simulink model "Retroacao_de_estados_2a_Lei_simulink"  (R2019a)
settings: Solver=ode45  StartTime=0.0  StopTime=2  RelTol=1e-3  EnableMultiTasking=on
values from neighbouring files (symbols this model uses):
  a = [-1 1; 1 -2]    [Ganhos_observador_de_estados.m]    (also in Observador_de_estados.m; Retroacao_de_estados_1a_Lei.m = [0 1; -40 -3]; Retroacao_de_estados_2a_Lei.m = [[0 1]; [0 -50]])
  b = [1;0]    [Ganhos_observador_de_estados.m]    (also in Observador_de_estados.m; Retroacao_de_estados_1a_Lei.m = [0 ; 40]; Retroacao_de_estados_2a_Lei.m = [0;1370])
  c = [1 0]    [Ganhos_observador_de_estados.m]    (also in Observador_de_estados.m; Retroacao_de_estados_2a_Lei.m = eye(2))
  d = 0    [Retroacao_de_estados_2a_Lei.m]
  K1 = K(1)    [Retroacao_de_estados_1a_Lei.m]    (also in Retroacao_de_estados_2a_Lei.m; Retroacao_de_estados_3a_Lei.m)
  K2 = K(2)    [Retroacao_de_estados_1a_Lei.m]    (also in Retroacao_de_estados_2a_Lei.m)
settings Model: Creator=Joao Paulo  LastModifiedBy=vinic
settings DataIOCC: LimitDataPoints=on  SaveFormat=Array  ReturnWorkspaceOutputs=off
settings OptimizationCC: ExpressionDepthLimit=2147483647  LifeSpan=inf
settings DebuggingCC: UnderspecifiedInitializationDetection=Classic  MergeDetectMultiDrivingBlocksExec=none  SolverPrmCheckMsg=warning  AllowSymbolicDim=off  StateNameClashWarn=warning  SFUnexpectedBacktrackingDiag=warning  SFNoUnconditionalDefaultTransitionDiag=warning  SFExecutionAtInitializationDiag=none  ArithmeticOperatorsInVariantConditions=warning
settings HardwareCC: ProdBitPerPointer=32  ProdBitPerSizeT=32  ProdBitPerPtrDiffT=32  ProdLargestAtomicFloat=None  ProdIntDivRoundTo=Undefined  ProdEndianess=Unspecified  ProdWordSize=32  ProdHWDeviceType=32-bit Generic
settings ModelReferenceCC: PropagateSignalLabelsOutOfModel=off
settings SFSimCC: SimUseLocalCustomCode=off
settings RTWCC: RTWUseLocalCustomCode=off
settings CodeAppCC: StateflowObjectComments=on
settings GRTTargetCC: TargetLangStandard=C89/C90 (ANSI)  GeneratePreprocessorConditionals=Disable all
settings ConfigComp: CovMetricSettings=dw  CovHtmlReporting=on  CovSaveCumulativeToWorkspaceVar=on  CovSaveSingleToWorkspaceVar=on  CovExternalEMLEnable=off

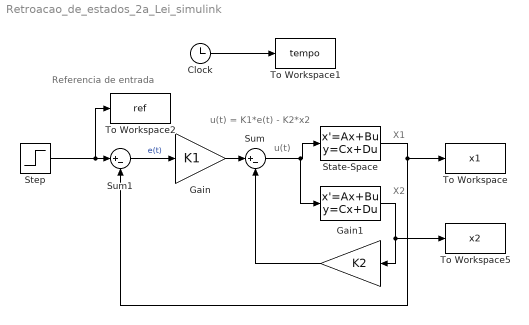
== system Retroacao_de_estados_2a_Lei_simulink ==
  note: Referencia de entrada
  note: u(t) = K1*e(t) - K2*x2
  note: u(t)
  note: X2
  note: X1
  " " : StateSpace  A=a  B=b  C=c(2,:)  D=d  InitialCondition=0
  Clock : Clock
  Gain : Gain  Gain=K1
  Gain1 : Gain  Gain=K2
  State-Space : StateSpace  A=a  B=b  C=c(1,:)  D=d  InitialCondition=0
  Step : Step  Time=0  SampleTime=0
  Sum : Sum  Inputs=|+-
  Sum1 : Sum  Inputs=|+-
  To Workspace : ToWorkspace  VariableName=x1  SampleTime=-1
  To Workspace1 : ToWorkspace  VariableName=tempo  SampleTime=-1
  To Workspace2 : ToWorkspace  VariableName=ref  SampleTime=-1
  To Workspace5 : ToWorkspace  VariableName=x2  SampleTime=-1
  wires:
  Sum/1 -> " "/1, State-Space/1
  Gain/1 -> Sum/1
  Gain1/1 -> Sum/2
  Step/1 -> To Workspace2/1, Sum1/1
  Clock/1 -> To Workspace1/1
  Sum1/1 -> Gain/1  "e(t)"
  State-Space/1 -> To Workspace/1, Sum1/2
  " "/1 -> To Workspace5/1, Gain1/1
